simulink library "libLeadingEdgeFlapDefCalc"  (R2020b)
settings: Solver=VariableStepAuto  StartTime=0.0  StopTime=10.0  RelTol=1e-3
undefined symbols (not defined in the file): outputs
settings Model: Creator=caatay  LastModifiedBy=caatay

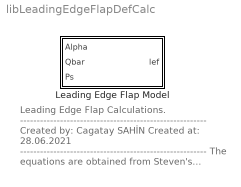
== system libLeadingEdgeFlapDefCalc ==
  note: Leading Edge Flap Calculations.
      | --------------------------------------------------------
      | Created by: Cagatay SAHİN
      | Created at: 28.06.2021
      | --------------------------------------------------------
      | The equations are obtained from
      | Steven's textbook.
      | The reference book can be found in
      | "references folder".
      | --------------------------------------------------------
      | for question:
      | cagataysahin44@gmail.com
  Leading Edge Flap Model : Subsystem  mask(Flight Control System Model - Leading Edge Flap Model){initAlphaDeg=-outputs.trim.states.alpha*180/pi}
      mask prompts: initAlphaDeg "Initial AoA in degree"
      mask help: Aircraft's leading edge flap deflection calculations. The model are obtained with using state and control information.
      mask Help:
      | This block is used for obtain leading edge flap deflection with using state and control inputs.
      | --------------------------------------------------------------------------------------------------------------------------------------------------
      | Input of the function:
      | 	alpha: Angle of attack (deg)
      | 	psta: Static Pressure (lb/ft^2)
      | 	qbar: Dynamic Presure (lb/ft^2)
      | Output of the function:
      | 	lef: Leading Edge Flap Deflection (deg)
      | --------------------------------------------------------------------------------------------------------------------------------------------------
      | All equations can be found in Steven's text book. Reference can be found in "literature" subfolder.
      | for question: "cagataysahin44@gmail.com"
      mask Display:
      | port_label('input',1,'\alpha','texmode','on');
      | port_label('input',2,'qbar','texmode','on');
      | port_label('input',3,'psta','texmode','on');
      | 
      | port_label('output',1,'\delta_{LEF_{act}}','texmode','on');

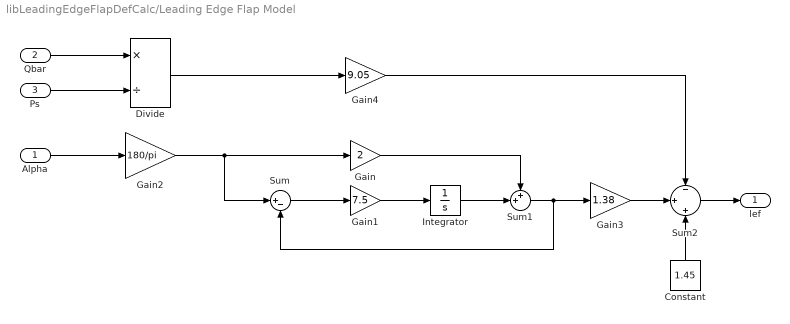
== system libLeadingEdgeFlapDefCalc/Leading Edge Flap Model ==
  Alpha : Inport
  Qbar : Inport  Port=2
  Ps : Inport  Port=3
  Constant : Constant  Value=1.45
  Divide : Product  Inputs=*/
  Gain : Gain  Gain=2
  Gain1 : Gain  Gain=7.5
  Gain2 : Gain  Gain=180/pi
  Gain3 : Gain  Gain=1.38
  Gain4 : Gain  Gain=9.05
  Integrator : Integrator  InitialCondition=initAlphaDeg
  Sum : Sum  Inputs=|+-
  Sum1 : Sum  Inputs=++|
  Sum2 : Sum  Inputs=-|+|+
  lef : Outport
  wires:
  Sum1/1 -> Sum/2, Gain3/1
  Gain4/1 -> Sum2/1
  Gain3/1 -> Sum2/2
  Gain/1 -> Sum1/1
  Constant/1 -> Sum2/3
  Integrator/1 -> Sum1/2
  Ps/1 -> Divide/2
  Gain2/1 -> Sum/1, Gain/1
  Sum/1 -> Gain1/1
  Gain1/1 -> Integrator/1
  Alpha/1 -> Gain2/1
  Divide/1 -> Gain4/1
  Sum2/1 -> lef/1
  Qbar/1 -> Divide/1
